simulink model "CDPRSim"  (R2023a)
settings: Solver=FixedStepAuto  StartTime=0.0  StopTime=inf  FixedStep=0.0001  RelTol=1e-3
values from neighbouring files (symbols this model uses):
  x11 = input('Enter x11 ')    [CDPRm.m]
  y11 = input('Enter y11 ')    [CDPRm.m]
undefined symbols (not defined in the file or in its folder): LBA, LTA, RBA, RTA
libraries: dspmathops x2, vrlib x1
(part 2 of 2)

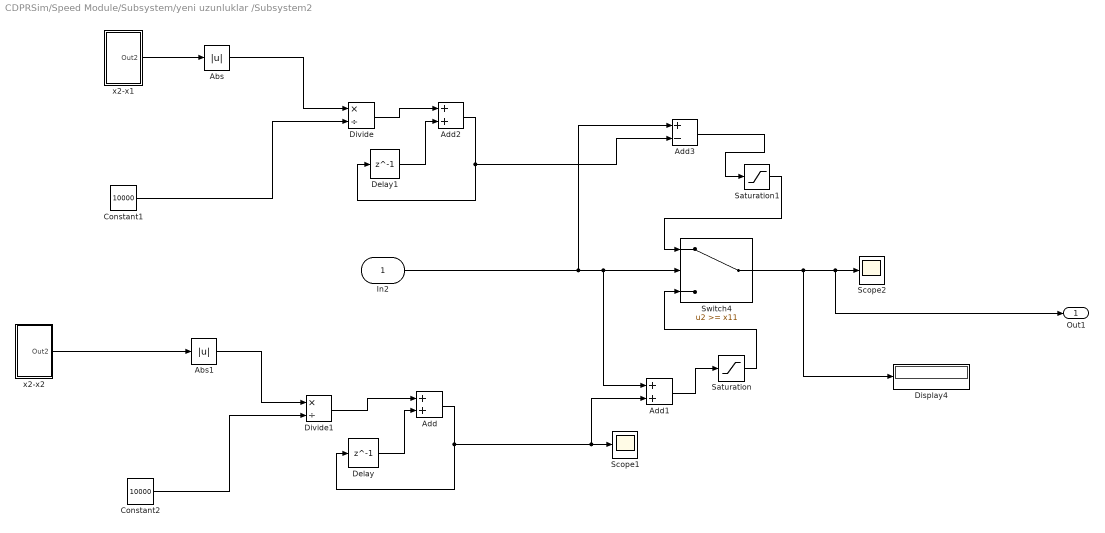
== system CDPRSim/Speed Module/Subsystem/yeni uzunluklar /Subsystem2 ==
  In2 : Inport
  Abs : Abs  SaturateOnIntegerOverflow=off
  Abs1 : Abs  SaturateOnIntegerOverflow=off
  Add : Sum
  Add1 : Sum
  Add2 : Sum
  Add3 : Sum  Inputs=+-
  Constant1 : Constant  Value=10000
  Constant2 : Constant  Value=10000
  Delay : Delay  DelayLength=1  InitialCondition=0
  Delay1 : Delay  DelayLength=1  InitialCondition=0
  Display4 : Display
  Divide : Product  Inputs=*/
  Divide1 : Product  Inputs=*/
  Saturation : Saturate  UpperLimit=x11  LowerLimit=0
  Saturation1 : Saturate  UpperLimit=1000  LowerLimit=x11
  Scope1 : Scope
  Scope2 : Scope
  Switch4 : Switch  Threshold=x11  SaturateOnIntegerOverflow=off  InputSameDT=off
  x2-x1 : Subsystem
  x2-x2 : Subsystem
  Out1 : Outport  VectorParamsAs1DForOutWhenUnconnected=off
  wires:
  Switch4/1 -> Display4/1, Out1/1, Scope2/1
  Divide1/1 -> Add/1
  In2/1 -> Add3/1, Add1/1, Switch4/2
  Delay/1 -> Add/2
  Add/1 -> Delay/1, Add1/2, Scope1/1
  Delay1/1 -> Add2/2
  Divide/1 -> Add2/1
  Add3/1 -> Saturation1/1
  Add2/1 -> Add3/2, Delay1/1
  Add1/1 -> Saturation/1
  Saturation/1 -> Switch4/3
  Saturation1/1 -> Switch4/1
  Abs/1 -> Divide/1
  x2-x1/1(Out2) -> Abs/1
  Constant1/1 -> Divide/2
  Abs1/1 -> Divide1/1
  x2-x2/1(Out2) -> Abs1/1
  Constant2/1 -> Divide1/2

== system CDPRSim/Speed Module/Left bottom hız /y value/Eski X/Triggered Subsystem4 ==
  In1 : Inport
  Trigger : TriggerPort  TriggerType=falling  VariantControl=Variant
  Out1 : Outport  VectorParamsAs1DForOutWhenUnconnected=off
  wires:
  In1/1 -> Out1/1

== system CDPRSim/Speed Module/Left bottom hız /y value/Subsystem1/x2-x1 ==
  Constant : Constant
  Display8 : Display
  Gain : Gain  Gain=x11
  Relational Operator4 : RelationalOperator  Operator===  OutDataTypeStr=boolean  RndMeth=Simplest  InputSameDT=off
  Sum5 : Sum  Inputs=|+-
  Triggered Subsystem4 : Subsystem  TreatAsAtomicUnit=on
  Unit Delay5 : UnitDelay  SampleTime=-1  HasFrameUpgradeWarning=on
  Out2 : Outport  VectorParamsAs1DForOutWhenUnconnected=off
  wires:
  Sum5/1 -> Out2/1, Display8/1
  Triggered Subsystem4/1(Out1) -> Sum5/2
  Unit Delay5/1 -> Relational Operator4/2, Triggered Subsystem4/1(In1)
  Gain/1 -> Sum5/1, Unit Delay5/1, Relational Operator4/1
  Relational Operator4/1 -> Triggered Subsystem4/Trigger
  Constant/1 -> Gain/1

== system CDPRSim/Speed Module/Left bottom hız /y value/Subsystem1/x2-x2 ==
  Constant1 : Constant
  Display8 : Display
  Gain : Gain  Gain=x11
  Relational Operator4 : RelationalOperator  Operator===  OutDataTypeStr=boolean  RndMeth=Simplest  InputSameDT=off
  Sum5 : Sum  Inputs=|+-
  Triggered Subsystem4 : Subsystem  TreatAsAtomicUnit=on
  Unit Delay5 : UnitDelay  SampleTime=-1  HasFrameUpgradeWarning=on
  Out2 : Outport  VectorParamsAs1DForOutWhenUnconnected=off
  wires:
  Sum5/1 -> Out2/1, Display8/1
  Triggered Subsystem4/1(Out1) -> Sum5/2
  Unit Delay5/1 -> Relational Operator4/2, Triggered Subsystem4/1(In1)
  Gain/1 -> Sum5/1, Unit Delay5/1, Relational Operator4/1
  Relational Operator4/1 -> Triggered Subsystem4/Trigger
  Constant1/1 -> Gain/1

== system CDPRSim/Speed Module/Left bottom hız /yeni uzunluklar /Eski X/Triggered Subsystem4 ==
  In1 : Inport
  Trigger : TriggerPort  TriggerType=falling  VariantControl=Variant
  Out1 : Outport  VectorParamsAs1DForOutWhenUnconnected=off
  wires:
  In1/1 -> Out1/1

== system CDPRSim/Speed Module/Left bottom hız /yeni uzunluklar /Subsystem2/x2-x1 ==
  Constant1 : Constant
  Display8 : Display
  Gain : Gain  Gain=x11
  Relational Operator4 : RelationalOperator  Operator===  OutDataTypeStr=boolean  RndMeth=Simplest  InputSameDT=off
  Sum5 : Sum  Inputs=|+-
  Triggered Subsystem4 : Subsystem  TreatAsAtomicUnit=on
  Unit Delay5 : UnitDelay  SampleTime=-1  HasFrameUpgradeWarning=on
  Out2 : Outport  VectorParamsAs1DForOutWhenUnconnected=off
  wires:
  Sum5/1 -> Out2/1, Display8/1
  Triggered Subsystem4/1(Out1) -> Sum5/2
  Unit Delay5/1 -> Relational Operator4/2, Triggered Subsystem4/1(In1)
  Gain/1 -> Sum5/1, Unit Delay5/1, Relational Operator4/1
  Relational Operator4/1 -> Triggered Subsystem4/Trigger
  Constant1/1 -> Gain/1

== system CDPRSim/Speed Module/Left bottom hız /yeni uzunluklar /Subsystem2/x2-x2 ==
  Constant1 : Constant
  Display8 : Display
  Gain : Gain  Gain=x11
  Relational Operator4 : RelationalOperator  Operator===  OutDataTypeStr=boolean  RndMeth=Simplest  InputSameDT=off
  Sum5 : Sum  Inputs=|+-
  Triggered Subsystem4 : Subsystem  TreatAsAtomicUnit=on
  Unit Delay5 : UnitDelay  SampleTime=-1  HasFrameUpgradeWarning=on
  Out2 : Outport  VectorParamsAs1DForOutWhenUnconnected=off
  wires:
  Sum5/1 -> Out2/1, Display8/1
  Triggered Subsystem4/1(Out1) -> Sum5/2
  Unit Delay5/1 -> Relational Operator4/2, Triggered Subsystem4/1(In1)
  Gain/1 -> Sum5/1, Unit Delay5/1, Relational Operator4/1
  Relational Operator4/1 -> Triggered Subsystem4/Trigger
  Constant1/1 -> Gain/1

== system CDPRSim/Speed Module/Subsystem/y value/Eski X/Triggered Subsystem4 ==
  In1 : Inport
  Trigger : TriggerPort  TriggerType=falling  VariantControl=Variant
  Out1 : Outport  VectorParamsAs1DForOutWhenUnconnected=off
  wires:
  In1/1 -> Out1/1

== system CDPRSim/Speed Module/Subsystem/y value/Subsystem2/x2-x1 ==
  Constant : Constant
  Constant2 : Constant
  Constant3 : Constant
  Display8 : Display
  Gain : Gain  Gain=x11
  Gain2 : Gain  Gain=1000
  Gain3 : Gain  Gain=70
  Relational Operator4 : RelationalOperator  Operator===  OutDataTypeStr=boolean  RndMeth=Simplest  InputSameDT=off
  Sum1 : Sum  Inputs=|+--
  Sum5 : Sum  Inputs=|+-
  Triggered Subsystem4 : Subsystem  TreatAsAtomicUnit=on
  Unit Delay5 : UnitDelay  SampleTime=-1  HasFrameUpgradeWarning=on
  Out2 : Outport  VectorParamsAs1DForOutWhenUnconnected=off
  wires:
  Sum5/1 -> Out2/1, Display8/1
  Triggered Subsystem4/1(Out1) -> Sum5/2
  Unit Delay5/1 -> Relational Operator4/2, Triggered Subsystem4/1(In1)
  Sum1/1 -> Sum5/1, Unit Delay5/1, Relational Operator4/1
  Relational Operator4/1 -> Triggered Subsystem4/Trigger
  Constant3/1 -> Gain3/1
  Gain3/1 -> Sum1/3
  Constant2/1 -> Gain/1
  Constant/1 -> Gain2/1
  Gain2/1 -> Sum1/1
  Gain/1 -> Sum1/2

== system CDPRSim/Speed Module/Subsystem/y value/Subsystem2/x2-x2 ==
  Constant : Constant
  Constant2 : Constant
  Constant3 : Constant
  Display8 : Display
  Gain : Gain  Gain=x11
  Gain2 : Gain  Gain=1000
  Gain3 : Gain  Gain=70
  Relational Operator4 : RelationalOperator  Operator===  OutDataTypeStr=boolean  RndMeth=Simplest  InputSameDT=off
  Sum1 : Sum  Inputs=|+--
  Sum5 : Sum  Inputs=|+-
  Triggered Subsystem4 : Subsystem  TreatAsAtomicUnit=on
  Unit Delay5 : UnitDelay  SampleTime=-1  HasFrameUpgradeWarning=on
  Out2 : Outport  VectorParamsAs1DForOutWhenUnconnected=off
  wires:
  Sum5/1 -> Out2/1, Display8/1
  Triggered Subsystem4/1(Out1) -> Sum5/2
  Unit Delay5/1 -> Relational Operator4/2, Triggered Subsystem4/1(In1)
  Sum1/1 -> Sum5/1, Unit Delay5/1, Relational Operator4/1
  Relational Operator4/1 -> Triggered Subsystem4/Trigger
  Constant3/1 -> Gain3/1
  Gain3/1 -> Sum1/3
  Constant2/1 -> Gain/1
  Constant/1 -> Gain2/1
  Gain2/1 -> Sum1/1
  Gain/1 -> Sum1/2

== system CDPRSim/Speed Module/Subsystem/yeni uzunluklar /Eski X/Triggered Subsystem4 ==
  In1 : Inport
  Trigger : TriggerPort  TriggerType=falling  VariantControl=Variant
  Out1 : Outport  VectorParamsAs1DForOutWhenUnconnected=off
  wires:
  In1/1 -> Out1/1

== system CDPRSim/Speed Module/Subsystem/yeni uzunluklar /Subsystem2/x2-x1 ==
  Constant : Constant
  Constant2 : Constant
  Constant3 : Constant
  Display8 : Display
  Gain : Gain  Gain=x11
  Gain2 : Gain  Gain=1000
  Gain3 : Gain  Gain=70
  Relational Operator4 : RelationalOperator  Operator===  OutDataTypeStr=boolean  RndMeth=Simplest  InputSameDT=off
  Sum1 : Sum  Inputs=|+--
  Sum5 : Sum  Inputs=|+-
  Triggered Subsystem4 : Subsystem  TreatAsAtomicUnit=on
  Unit Delay5 : UnitDelay  SampleTime=-1  HasFrameUpgradeWarning=on
  Out2 : Outport  VectorParamsAs1DForOutWhenUnconnected=off
  wires:
  Sum5/1 -> Out2/1, Display8/1
  Triggered Subsystem4/1(Out1) -> Sum5/2
  Unit Delay5/1 -> Relational Operator4/2, Triggered Subsystem4/1(In1)
  Sum1/1 -> Sum5/1, Relational Operator4/1, Unit Delay5/1
  Relational Operator4/1 -> Triggered Subsystem4/Trigger
  Constant3/1 -> Gain3/1
  Gain3/1 -> Sum1/3
  Constant2/1 -> Gain/1
  Constant/1 -> Gain2/1
  Gain2/1 -> Sum1/1
  Gain/1 -> Sum1/2

== system CDPRSim/Speed Module/Subsystem/yeni uzunluklar /Subsystem2/x2-x2 ==
  Constant : Constant
  Constant2 : Constant
  Constant3 : Constant
  Display8 : Display
  Gain : Gain  Gain=x11
  Gain2 : Gain  Gain=1000
  Gain3 : Gain  Gain=70
  Relational Operator4 : RelationalOperator  Operator===  OutDataTypeStr=boolean  RndMeth=Simplest  InputSameDT=off
  Sum1 : Sum  Inputs=|+--
  Sum5 : Sum  Inputs=|+-
  Triggered Subsystem4 : Subsystem  TreatAsAtomicUnit=on
  Unit Delay5 : UnitDelay  SampleTime=-1  HasFrameUpgradeWarning=on
  Out2 : Outport  VectorParamsAs1DForOutWhenUnconnected=off
  wires:
  Sum5/1 -> Out2/1, Display8/1
  Triggered Subsystem4/1(Out1) -> Sum5/2
  Unit Delay5/1 -> Relational Operator4/2, Triggered Subsystem4/1(In1)
  Sum1/1 -> Sum5/1, Relational Operator4/1, Unit Delay5/1
  Relational Operator4/1 -> Triggered Subsystem4/Trigger
  Constant3/1 -> Gain3/1
  Gain3/1 -> Sum1/3
  Constant2/1 -> Gain/1
  Constant/1 -> Gain2/1
  Gain2/1 -> Sum1/1
  Gain/1 -> Sum1/2

== system CDPRSim/Speed Module/Left bottom hız /y value/Subsystem1/x2-x1/Triggered Subsystem4 ==
  In1 : Inport
  Trigger : TriggerPort  TriggerType=falling  VariantControl=Variant
  Out1 : Outport  VectorParamsAs1DForOutWhenUnconnected=off
  wires:
  In1/1 -> Out1/1

== system CDPRSim/Speed Module/Left bottom hız /y value/Subsystem1/x2-x2/Triggered Subsystem4 ==
  In1 : Inport
  Trigger : TriggerPort  TriggerType=falling  VariantControl=Variant
  Out1 : Outport  VectorParamsAs1DForOutWhenUnconnected=off
  wires:
  In1/1 -> Out1/1

== system CDPRSim/Speed Module/Left bottom hız /yeni uzunluklar /Subsystem2/x2-x1/Triggered Subsystem4 ==
  In1 : Inport
  Trigger : TriggerPort  TriggerType=falling  VariantControl=Variant
  Out1 : Outport  VectorParamsAs1DForOutWhenUnconnected=off
  wires:
  In1/1 -> Out1/1

== system CDPRSim/Speed Module/Left bottom hız /yeni uzunluklar /Subsystem2/x2-x2/Triggered Subsystem4 ==
  In1 : Inport
  Trigger : TriggerPort  TriggerType=falling  VariantControl=Variant
  Out1 : Outport  VectorParamsAs1DForOutWhenUnconnected=off
  wires:
  In1/1 -> Out1/1

== system CDPRSim/Speed Module/Subsystem/y value/Subsystem2/x2-x1/Triggered Subsystem4 ==
  In1 : Inport
  Trigger : TriggerPort  TriggerType=falling  VariantControl=Variant
  Out1 : Outport  VectorParamsAs1DForOutWhenUnconnected=off
  wires:
  In1/1 -> Out1/1

== system CDPRSim/Speed Module/Subsystem/y value/Subsystem2/x2-x2/Triggered Subsystem4 ==
  In1 : Inport
  Trigger : TriggerPort  TriggerType=falling  VariantControl=Variant
  Out1 : Outport  VectorParamsAs1DForOutWhenUnconnected=off
  wires:
  In1/1 -> Out1/1

== system CDPRSim/Speed Module/Subsystem/yeni uzunluklar /Subsystem2/x2-x1/Triggered Subsystem4 ==
  In1 : Inport
  Trigger : TriggerPort  TriggerType=falling  VariantControl=Variant
  Out1 : Outport  VectorParamsAs1DForOutWhenUnconnected=off
  wires:
  In1/1 -> Out1/1

== system CDPRSim/Speed Module/Subsystem/yeni uzunluklar /Subsystem2/x2-x2/Triggered Subsystem4 ==
  In1 : Inport
  Trigger : TriggerPort  TriggerType=falling  VariantControl=Variant
  Out1 : Outport  VectorParamsAs1DForOutWhenUnconnected=off
  wires:
  In1/1 -> Out1/1
